simulink model "Model_UAV"  (R2023b)
settings: Solver=VariableStepAuto  StartTime=0.0  StopTime=10.0  RelTol=1e-3
values from neighbouring files (symbols this model uses):
  Area = 0.1    [Parameters.m]
  C_d = 1.05    [Parameters.m]
  cg_pos = [0.03 0 0.7]    [Parameters.m]
  ct_pos = [0 0 0.2]    [Parameters.m]
  Mass = 2    [Parameters.m]
libraries: simulink_extras x2, shared6dof x1, vrlib x1, matrix_library x1, sharedtransform x1
settings Model: Creator=zbyss  LastModifiedBy=zbyss

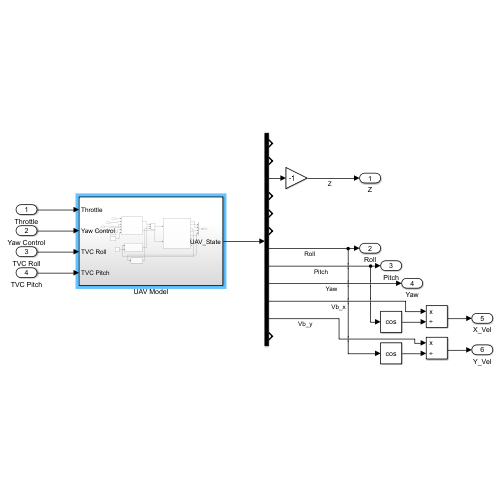
[thumbnail: Simulink's stored preview of the top-level diagram]
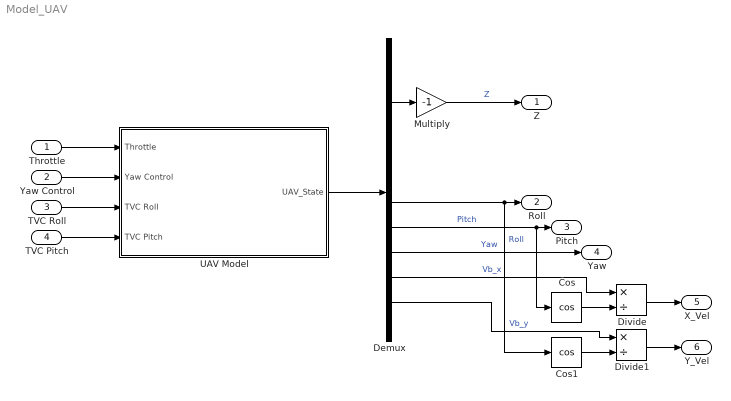
== system Model_UAV ==
  Throttle : Inport
  Yaw Control : Inport  Port=2
  TVC Roll : Inport  Port=3
  TVC Pitch : Inport  Port=4
  Cos : Trigonometry  Operator=cos
  Cos1 : Trigonometry  Operator=cos
  Demux : Demux  Outputs=12
  Divide : Product  Inputs=*/
  Divide1 : Product  Inputs=*/
  Multiply : Gain  Gain=-1
  UAV Model : Subsystem
  Z : Outport
  Roll : Outport  Port=2
  Pitch : Outport  Port=3
  Yaw : Outport  Port=4
  X_Vel : Outport  Port=5
  Y_Vel : Outport  Port=6
  wires:
  Demux/8 -> Cos/1, Pitch/1  "Pitch"
  UAV Model/1(UAV_State) -> Demux/1
  Demux/10 -> Divide/1  "Vb_x"
  Demux/7 -> Cos1/1, Roll/1  "Roll"
  Demux/11 -> Divide1/1  "Vb_y"
  Multiply/1 -> Z/1  "Z"
  Demux/3 -> Multiply/1
  Demux/9 -> Yaw/1  "Yaw"
  Cos/1 -> Divide/2
  Cos1/1 -> Divide1/2
  Divide/1 -> X_Vel/1
  Divide1/1 -> Y_Vel/1
  Throttle/1 -> UAV Model/1(Throttle)
  Yaw Control/1 -> UAV Model/2(Yaw Control)
  TVC Roll/1 -> UAV Model/3(TVC Roll)
  TVC Pitch/1 -> UAV Model/4(TVC Pitch)

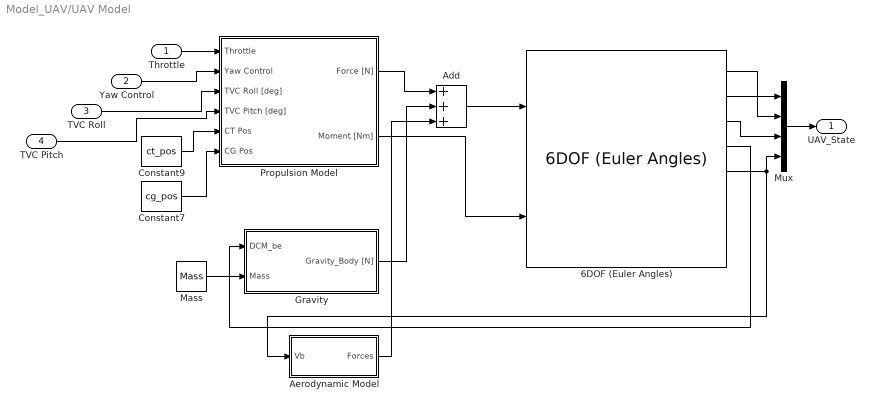
== system Model_UAV/UAV Model ==
  Throttle : Inport
  Yaw Control : Inport  Port=2
  TVC Roll : Inport  Port=3
  TVC Pitch : Inport  Port=4
  6DOF (Euler Angles) : shared6dof/6DOF (Euler Angles)  units=Metric (MKS)  mtype=Fixed  rep=Euler Angles  xme_0=[0 0 0]  Vm_0=[0 0 0]  eul_0=[0 0 0]  pm_0=[0 0 0]  mass_0=Mass  mass_e=0.5  mass_f=2.0  inertia=eye(3)  inertia_e=eye(3)  inertia_f=2*eye(3)  k_quat=1.0  vre_flag=on  abi_flag=off  aMode=0  xme_statename=''  Vm_statename=''  eul_statename=''  quat_statename=''  pm_statename=''  mass_statename=''
  Add : Sum  Inputs=+++
  Aerodynamic Model : Subsystem
  Constant7 : Constant  Value=cg_pos
  Constant9 : Constant  Value=ct_pos
  Gravity : Subsystem
  Mass : Constant  Value=Mass
  Mux : Mux
  Propulsion Model : Subsystem
  UAV_State : Outport
  wires:
  Propulsion Model/1(Force [N]) -> Add/1
  Add/1 -> 6DOF (Euler Angles)/1
  TVC Roll/1 -> Propulsion Model/3(TVC Roll [deg])
  Throttle/1 -> Propulsion Model/1(Throttle)
  Gravity/1(Gravity_Body [N]) -> Add/2
  Propulsion Model/2(Moment [Nm]) -> 6DOF (Euler Angles)/2
  Constant9/1 -> Propulsion Model/5(CT Pos)
  Constant7/1 -> Propulsion Model/6(CG Pos)
  Mass/1 -> Gravity/2(Mass)
  6DOF (Euler Angles)/4 -> Gravity/1(DCM_be)
  Yaw Control/1 -> Propulsion Model/2(Yaw Control)
  6DOF (Euler Angles)/3 -> Mux/3
  6DOF (Euler Angles)/2 -> Mux/1
  Mux/1 -> UAV_State/1
  TVC Pitch/1 -> Propulsion Model/4(TVC Pitch [deg])
  6DOF (Euler Angles)/1 -> Mux/2
  6DOF (Euler Angles)/5 -> Aerodynamic Model/1(Vb), Mux/4
  Aerodynamic Model/1(Forces) -> Add/3

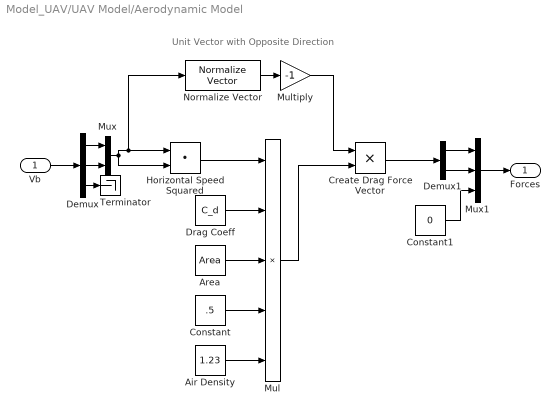
== system Model_UAV/UAV Model/Aerodynamic Model ==
  note: Unit Vector with Opposite Direction
  Vb : Inport
  Air Density : Constant  Value=1.23
  Area : Constant  Value=Area
  Constant : Constant  Value=.5
  Constant1 : Constant  Value=0
  Create Drag Force Vector : Product  Inputs=**
  Demux : Demux  Outputs=3
  Demux1 : Demux  Outputs=2
  Drag Coeff : Constant  Value=C_d
  Horizontal Speed Squared : DotProduct  OutDataTypeStr=Inherit: Inherit via internal rule
  Mul : Product  Inputs=*****
  Multiply : Gain  Gain=-1
  Mux : Mux  Inputs=2
  Mux1 : Mux  Inputs=3
  Normalize Vector : vrlib/Utilities/Normalize Vector  maxzero=0
  Terminator : Terminator
  Forces : Outport
  wires:
  Vb/1 -> Demux/1
  Demux/3 -> Terminator/1
  Demux/1 -> Mux/1
  Demux/2 -> Mux/2
  Normalize Vector/1 -> Multiply/1
  Mux/1 -> Horizontal Speed Squared/2, Normalize Vector/1, Horizontal Speed Squared/1
  Horizontal Speed Squared/1 -> Mul/1
  Drag Coeff/1 -> Mul/2
  Area/1 -> Mul/3
  Constant/1 -> Mul/4
  Air Density/1 -> Mul/5
  Multiply/1 -> Create Drag Force Vector/1
  Mul/1 -> Create Drag Force Vector/2
  Mux1/1 -> Forces/1
  Demux1/1 -> Mux1/1
  Demux1/2 -> Mux1/2
  Create Drag Force Vector/1 -> Demux1/1
  Constant1/1 -> Mux1/3

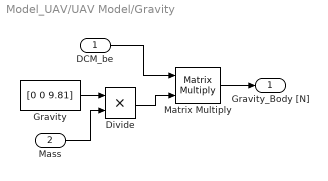
== system Model_UAV/UAV Model/Gravity ==
  DCM_be : Inport
  Mass : Inport  Port=2
  Divide : Product  Inputs=**
  Gravity : Constant  Value=[0 0 9.81]
  Matrix Multiply : Product  Multiplication=Matrix(*)
  Gravity_Body [N] : Outport
  wires:
  Matrix Multiply/1 -> Gravity_Body [N]/1
  DCM_be/1 -> Matrix Multiply/1
  Gravity/1 -> Divide/1
  Divide/1 -> Matrix Multiply/2
  Mass/1 -> Divide/2

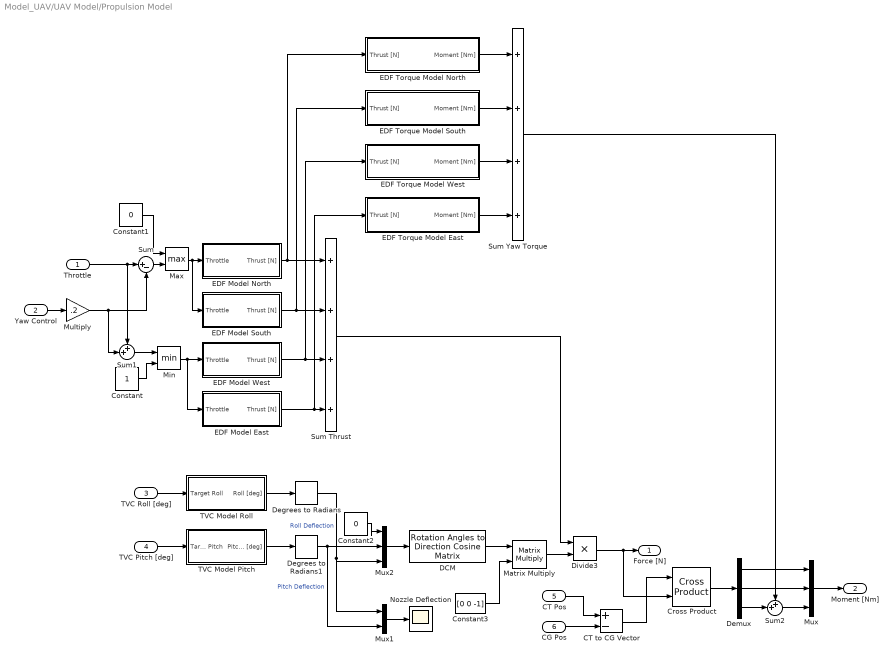
== system Model_UAV/UAV Model/Propulsion Model ==
  Throttle : Inport
  Yaw Control : Inport  Port=2
  TVC Roll [deg] : Inport  Port=3
  TVC Pitch [deg] : Inport  Port=4
  CT Pos : Inport  Port=5
  CG Pos : Inport  Port=6
  CT to CG Vector : Sum  Inputs=+-
  Constant : Constant
  Constant1 : Constant  Value=0
  Constant2 : Constant  Value=0
  Constant3 : Constant  Value=[0 0 -1]
  Cross Product : matrix_library/Cross Product
  DCM : sharedtransform/Rotation Angles to Direction Cosine Matrix  rotationOrder=ZYX  aMode=aMode
  Degrees to Radians : simulink_extras/Transformations/Degrees to Radians
  Degrees to Radians1 : simulink_extras/Transformations/Degrees to Radians
  Demux : Demux  Outputs=3
  Divide3 : Product  Inputs=**
  EDF Model East : Subsystem
  EDF Model North : Subsystem
  EDF Model South : Subsystem
  EDF Model West : Subsystem
  EDF Torque Model East : Subsystem
  EDF Torque Model North : Subsystem
  EDF Torque Model South : Subsystem
  EDF Torque Model West : Subsystem
  Matrix Multiply : Product  Multiplication=Matrix(*)
  Max : MinMax  Function=max  Inputs=2
  Min : MinMax  Inputs=2
  Multiply : Gain  Gain=.2
  Mux : Mux  Inputs=3
  Mux1 : Mux  Inputs=2
  Mux2 : Mux  Inputs=3
  Nozzle Deflection : Scope
  Sum : Sum  Inputs=|+-
  Sum Thrust : Sum  Inputs=++++
  Sum Yaw Torque : Sum  Inputs=++++
  Sum1 : Sum  Inputs=++|
  Sum2 : Sum  Inputs=++|
  TVC Model Pitch : Subsystem
  TVC Model Roll : Subsystem
  Force [N] : Outport
  Moment [Nm] : Outport  Port=2
  wires:
  TVC Roll [deg]/1 -> TVC Model Roll/1(Target Roll)
  EDF Model West/1(Thrust [N]) -> EDF Torque Model West/1(Thrust [N]), Sum Thrust/3
  EDF Model South/1(Thrust [N]) -> EDF Torque Model South/1(Thrust [N]), Sum Thrust/2
  EDF Model North/1(Thrust [N]) -> EDF Torque Model North/1(Thrust [N]), Sum Thrust/1
  EDF Model East/1(Thrust [N]) -> EDF Torque Model East/1(Thrust [N]), Sum Thrust/4
  TVC Pitch [deg]/1 -> TVC Model Pitch/1(Target Pitch)
  TVC Model Roll/1(Roll [deg]) -> Degrees to Radians/1
  TVC Model Pitch/1(Pitch [deg]) -> Degrees to Radians1/1
  Degrees to Radians/1 -> Mux1/1, Mux2/3  "Roll Deflection"
  Degrees to Radians1/1 -> Mux1/2, Mux2/2  "Pitch Deflection"
  Divide3/1 -> Cross Product/2, Force [N]/1
  Sum Thrust/1 -> Divide3/1
  Mux/1 -> Moment [Nm]/1
  EDF Torque Model North/1(Moment [Nm]) -> Sum Yaw Torque/1
  EDF Torque Model South/1(Moment [Nm]) -> Sum Yaw Torque/2
  EDF Torque Model West/1(Moment [Nm]) -> Sum Yaw Torque/3
  EDF Torque Model East/1(Moment [Nm]) -> Sum Yaw Torque/4
  Yaw Control/1 -> Multiply/1
  Multiply/1 -> Sum1/2, Sum/2
  Throttle/1 -> Sum/1, Sum1/1
  Min/1 -> EDF Model East/1(Throttle), EDF Model West/1(Throttle)
  Sum1/1 -> Min/1
  Constant/1 -> Min/2
  Max/1 -> EDF Model South/1(Throttle), EDF Model North/1(Throttle)
  Sum/1 -> Max/2
  Constant1/1 -> Max/1
  Mux1/1 -> Nozzle Deflection/1
  Mux2/1 -> DCM/1
  Constant2/1 -> Mux2/1
  DCM/1 -> Matrix Multiply/1
  Constant3/1 -> Matrix Multiply/2
  Matrix Multiply/1 -> Divide3/2
  CG Pos/1 -> CT to CG Vector/2
  CT Pos/1 -> CT to CG Vector/1
  CT to CG Vector/1 -> Cross Product/1
  Cross Product/1 -> Demux/1
  Demux/1 -> Mux/1
  Demux/2 -> Mux/2
  Demux/3 -> Sum2/2
  Sum2/1 -> Mux/3
  Sum Yaw Torque/1 -> Sum2/1

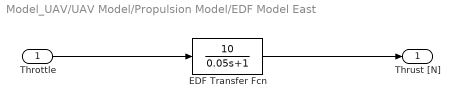
== system Model_UAV/UAV Model/Propulsion Model/EDF Model East ==
  Throttle : Inport
  EDF Transfer Fcn : TransferFcn  Numerator=[10]  Denominator=[0.05 1]
  Thrust [N] : Outport
  wires:
  Throttle/1 -> EDF Transfer Fcn/1
  EDF Transfer Fcn/1 -> Thrust [N]/1

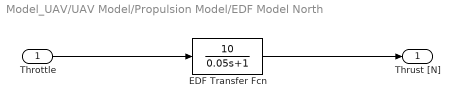
== system Model_UAV/UAV Model/Propulsion Model/EDF Model North ==
  Throttle : Inport
  EDF Transfer Fcn : TransferFcn  Numerator=[10]  Denominator=[0.05 1]
  Thrust [N] : Outport
  wires:
  Throttle/1 -> EDF Transfer Fcn/1
  EDF Transfer Fcn/1 -> Thrust [N]/1

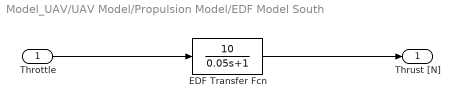
== system Model_UAV/UAV Model/Propulsion Model/EDF Model South ==
  Throttle : Inport
  EDF Transfer Fcn : TransferFcn  Numerator=[10]  Denominator=[0.05 1]
  Thrust [N] : Outport
  wires:
  Throttle/1 -> EDF Transfer Fcn/1
  EDF Transfer Fcn/1 -> Thrust [N]/1

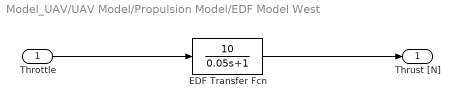
== system Model_UAV/UAV Model/Propulsion Model/EDF Model West ==
  Throttle : Inport
  EDF Transfer Fcn : TransferFcn  Numerator=[10]  Denominator=[0.05 1]
  Thrust [N] : Outport
  wires:
  Throttle/1 -> EDF Transfer Fcn/1
  EDF Transfer Fcn/1 -> Thrust [N]/1

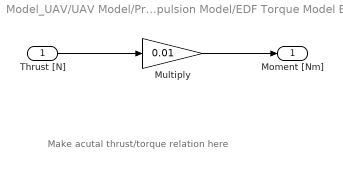
== system Model_UAV/UAV Model/Propulsion Model/EDF Torque Model East ==
  note: Make acutal thrust/torque relation here
  Thrust [N] : Inport
  Multiply : Gain  Gain=0.01
  Moment [Nm] : Outport
  wires:
  Thrust [N]/1 -> Multiply/1
  Multiply/1 -> Moment [Nm]/1

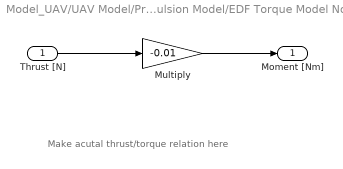
== system Model_UAV/UAV Model/Propulsion Model/EDF Torque Model North ==
  note: Make acutal thrust/torque relation here
  Thrust [N] : Inport
  Multiply : Gain  Gain=-0.01
  Moment [Nm] : Outport
  wires:
  Thrust [N]/1 -> Multiply/1
  Multiply/1 -> Moment [Nm]/1

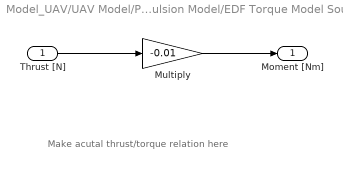
== system Model_UAV/UAV Model/Propulsion Model/EDF Torque Model South ==
  note: Make acutal thrust/torque relation here
  Thrust [N] : Inport
  Multiply : Gain  Gain=-0.01
  Moment [Nm] : Outport
  wires:
  Thrust [N]/1 -> Multiply/1
  Multiply/1 -> Moment [Nm]/1

== system Model_UAV/UAV Model/Propulsion Model/EDF Torque Model West ==
  note: Make acutal thrust/torque relation here
  Thrust [N] : Inport
  Multiply : Gain  Gain=0.01
  Moment [Nm] : Outport
  wires:
  Thrust [N]/1 -> Multiply/1
  Multiply/1 -> Moment [Nm]/1

== system Model_UAV/UAV Model/Propulsion Model/TVC Model Pitch ==
  Target Pitch : Inport
  Gimball Pitch Transfer Fcn : TransferFcn  Denominator=[0.05 1]
  Pitch [deg] : Outport
  wires:
  Target Pitch/1 -> Gimball Pitch Transfer Fcn/1
  Gimball Pitch Transfer Fcn/1 -> Pitch [deg]/1

== system Model_UAV/UAV Model/Propulsion Model/TVC Model Roll ==
  Target Roll : Inport
  Gimball Roll Transfer Fcn : TransferFcn  Denominator=[0.05 1]
  Roll [deg] : Outport
  wires:
  Target Roll/1 -> Gimball Roll Transfer Fcn/1
  Gimball Roll Transfer Fcn/1 -> Roll [deg]/1
